simulink model "ltslqgkalmanservo"  (Simulink 7.8)
settings: Solver=ode1  StartTime=0.0  StopTime=stoptime  FixedStep=(1/10000)  RelTol=1e-3
values from neighbouring files (symbols this model uses):
  Apaug = [Ap -Bp*Kpmcv; Kpf*Cp Ap-Kpf*Cp-Bp*Kpmcv]    [main.m]
  Ayaug = [Ayaw -Byaw*Kymcv; Kyf*Cyaw Ayaw-Kyf*Cyaw-Byaw*Kymcv]    [main.m]
  Bpaug = [Bp Gp zeros(4,1);Bp zeros(4,1) Kpf]    [main.m]
  Byaug = [Byaw Gyaw zeros(4,1);Byaw zeros(4,1) Kyf]    [main.m]
  Cpaug = eye(8,8)    [main.m]
  Cyaug = eye(8,8)    [main.m]
  Dpaug = zeros(8,3)    [main.m]
  dt = 0.0001    [main.m]
  Dyaug = zeros(8,3)    [main.m]
  V = (1e-5)*eye(mx)    [KalmanEstimator.m]    (also in main.m)
  W = (1e-3)*eye(ny)    [KalmanEstimator.m]    (also in main.m = (1e-4)*eye(ny))
undefined symbols (not defined in the file or in its folder): clock, Kpmcv, Kymcv
settings Model: Creator=Firdous  LastModifiedBy=Firdous
settings DataIOCC: LimitDataPoints=off  SaveState=on

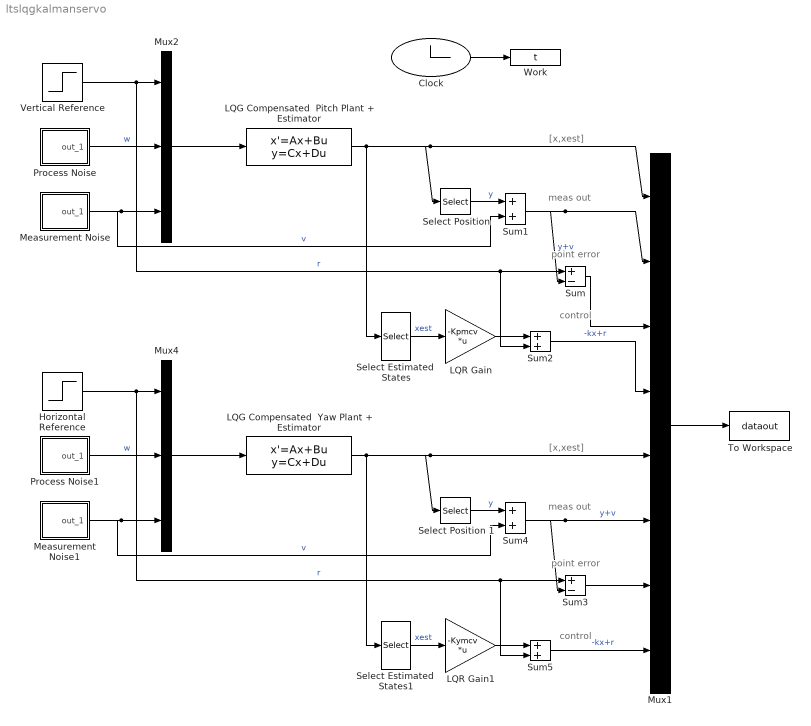
== system ltslqgkalmanservo ==
  note: control
  note: point
      | error
  note: meas
      | out
  note: [x,xest]
  note: control
  note: point
      | error
  note: meas
      | out
  note: [x,xest]
  Clock : Clock
  Horizontal Reference : Step  Time=0  After=15.15  SampleTime=0
  LQG Compensated  Pitch Plant + Estimator : StateSpace  A=Apaug  B=Bpaug  C=Cpaug  D=Dpaug  X0=[2 0 0 0 2 0 0 0]
  LQG Compensated  Yaw Plant + Estimator : StateSpace  A=Ayaug  B=Byaug  C=Cyaug  D=Dyaug  X0=[2 0 0 0 2 0 0 0]
  LQR Gain : Gain  Gain=-Kpmcv  Multiplication=Matrix(K*u) (u vector)
  LQR Gain1 : Gain  Gain=-Kymcv  Multiplication=Matrix(K*u) (u vector)
  Measurement Noise : Subsystem  mask(Continuous White Noise.){Cov=V, Ts=dt, seed=round(100*sum(clock))}
      mask prompts: Cov "Noise Variance:"; Ts "Sample Time:"
      mask help:
      | White noise for continuous (s-domain) systems.
      | Band-limited using zero-order-hold.
      mask Help: Implemented using white noise into Zero Order Hold block. For faster simulation set sample time to highest value possible but in accordance with the fastest dynamics of system.
      mask Display: plot(1:20,rand(size(1:20)))
  Measurement Noise1 : Subsystem  mask(Continuous White Noise.){Cov=V, Ts=dt, seed=round(100*sum(clock))}
      mask prompts: Cov "Noise Variance:"; Ts "Sample Time:"
      mask help:
      | White noise for continuous (s-domain) systems.
      | Band-limited using zero-order-hold.
      mask Help: Implemented using white noise into Zero Order Hold block. For faster simulation set sample time to highest value possible but in accordance with the fastest dynamics of system.
      mask Display: plot(1:20,rand(size(1:20)))
  Mux1 : Mux  Inputs=8
  Mux2 : Mux  Inputs=3
  Mux4 : Mux  Inputs=3
  Process Noise : Subsystem  mask(Continuous White Noise.){Cov=W, Ts=dt, seed=round(100*sum(clock))}
      mask prompts: Cov "Noise Variance:"; Ts "Sample Time:"
      mask help:
      | White noise for continuous (s-domain) systems.
      | Band-limited using zero-order-hold.
      mask Help: Implemented using white noise into Zero Order Hold block. For faster simulation set sample time to highest value possible but in accordance with the fastest dynamics of system.
      mask Display: plot(1:20,rand(size(1:20)))
  Process Noise1 : Subsystem  mask(Continuous White Noise.){Cov=W, Ts=dt, seed=round(100*sum(clock))}
      mask prompts: Cov "Noise Variance:"; Ts "Sample Time:"
      mask help:
      | White noise for continuous (s-domain) systems.
      | Band-limited using zero-order-hold.
      mask Help: Implemented using white noise into Zero Order Hold block. For faster simulation set sample time to highest value possible but in accordance with the fastest dynamics of system.
      mask Display: plot(1:20,rand(size(1:20)))
  Select Estimated  States : Selector  InputPortWidth=8  IndexOptions=Index vector (dialog)  Indices=[5,6,7,8]  OutputSizes=1
  Select Estimated  States1 : Selector  InputPortWidth=8  IndexOptions=Index vector (dialog)  Indices=[5,6,7,8]  OutputSizes=1
  "Select Position " : Selector  InputPortWidth=8  IndexOptions=Index vector (dialog)  Indices=[1]  OutputSizes=1
  Select Position 1 : Selector  InputPortWidth=8  IndexOptions=Index vector (dialog)  Indices=[1]  OutputSizes=1
  Sum : Sum  Inputs=+-
  Sum{1..2,4..5} (4 alike) : Sum
  Sum3 : Sum  Inputs=+-
  To Workspace : ToWorkspace  VariableName=dataout  SampleTime=-1  SaveFormat=Array
  Vertical Reference : Step  Time=0  After=15.15  SampleTime=0
  Work : ToWorkspace  VariableName=t  SaveFormat=Array
      settings: MaxDataPoints=stoptime
  wires:
  Mux2/1 -> LQG Compensated  Pitch Plant + Estimator/1
  Select Estimated  States/1 -> LQR Gain/1  "xest"
  LQR Gain/1 -> Sum2/1
  Vertical Reference/1 -> Mux2/1, Sum/1, Sum2/2  "r"
  Process Noise/1(out_1) -> Mux2/2  "w"
  Measurement Noise/1(out_1) -> Mux2/3, Sum1/2  "v"
  "Select Position "/1 -> Sum1/1  "y"
  LQG Compensated  Pitch Plant + Estimator/1 -> Mux1/1, "Select Position "/1, Select Estimated  States/1
  Sum1/1 -> Mux1/2, Sum/2  "y+v"
  Sum/1 -> Mux1/3
  Sum2/1 -> Mux1/4  "-kx+r"
  Mux4/1 -> LQG Compensated  Yaw Plant + Estimator/1
  Select Estimated  States1/1 -> LQR Gain1/1  "xest"
  LQR Gain1/1 -> Sum5/1
  Horizontal Reference/1 -> Mux4/1, Sum3/1, Sum5/2  "r"
  Process Noise1/1(out_1) -> Mux4/2  "w"
  Measurement Noise1/1(out_1) -> Mux4/3, Sum4/2  "v"
  Select Position 1/1 -> Sum4/1  "y"
  LQG Compensated  Yaw Plant + Estimator/1 -> Select Position 1/1, Mux1/5, Select Estimated  States1/1
  Sum4/1 -> Sum3/2, Mux1/6  "y+v"
  Sum3/1 -> Mux1/7
  Sum5/1 -> Mux1/8  "-kx+r"
  Mux1/1 -> To Workspace/1
  Clock/1 -> Work/1

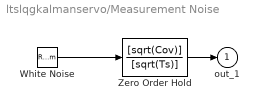
== system ltslqgkalmanservo/Measurement Noise ==
  White Noise : RandomNumber  Seed=seed  SampleTime=dt
  Zero Order Hold : DiscreteTransferFcn  Numerator=[sqrt(Cov)]  Denominator=[sqrt(Ts)]  SampleTime=Ts
  out_1 : Outport
  wires:
  Zero Order Hold/1 -> out_1/1
  White Noise/1 -> Zero Order Hold/1

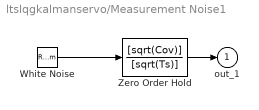
== system ltslqgkalmanservo/Measurement Noise1 ==
  White Noise : RandomNumber  Seed=seed  SampleTime=dt
  Zero Order Hold : DiscreteTransferFcn  Numerator=[sqrt(Cov)]  Denominator=[sqrt(Ts)]  SampleTime=Ts
  out_1 : Outport
  wires:
  Zero Order Hold/1 -> out_1/1
  White Noise/1 -> Zero Order Hold/1

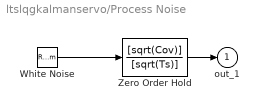
== system ltslqgkalmanservo/Process Noise ==
  White Noise : RandomNumber  Seed=seed  SampleTime=dt
  Zero Order Hold : DiscreteTransferFcn  Numerator=[sqrt(Cov)]  Denominator=[sqrt(Ts)]  SampleTime=Ts
  out_1 : Outport
  wires:
  Zero Order Hold/1 -> out_1/1
  White Noise/1 -> Zero Order Hold/1

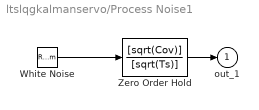
== system ltslqgkalmanservo/Process Noise1 ==
  White Noise : RandomNumber  Seed=seed  SampleTime=dt
  Zero Order Hold : DiscreteTransferFcn  Numerator=[sqrt(Cov)]  Denominator=[sqrt(Ts)]  SampleTime=Ts
  out_1 : Outport
  wires:
  Zero Order Hold/1 -> out_1/1
  White Noise/1 -> Zero Order Hold/1
